simulink model "UAV_Hover_Sim_Soln"  (R2025a)
settings: Solver=VariableStepAuto  StartTime=0.0  StopTime=inf  RelTol=1e-3
undefined symbols (not defined in the file): quad_m, W
libraries: slpidlib x1, aerolibanimutils x1, uavutilslib x1, aerolibobsolete x1
settings Model: Creator=Aorus PC  LastModifiedBy=esmithzb
settings OptimizationCC: ReuseModelBlockBuffer=off
settings DebuggingCC: UnderspecifiedInitializationDetection=Classic  MergeDetectMultiDrivingBlocksExec=none
settings ModelReferenceCC: PropagateSignalLabelsOutOfModel=off
settings RTWCC: GPUComputeCapability=3.5

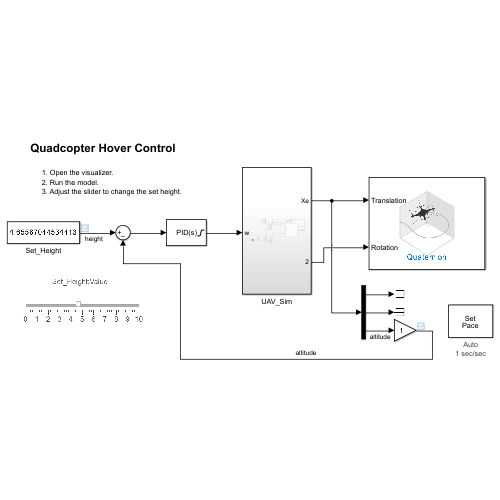
[thumbnail: Simulink's stored preview of the top-level diagram]
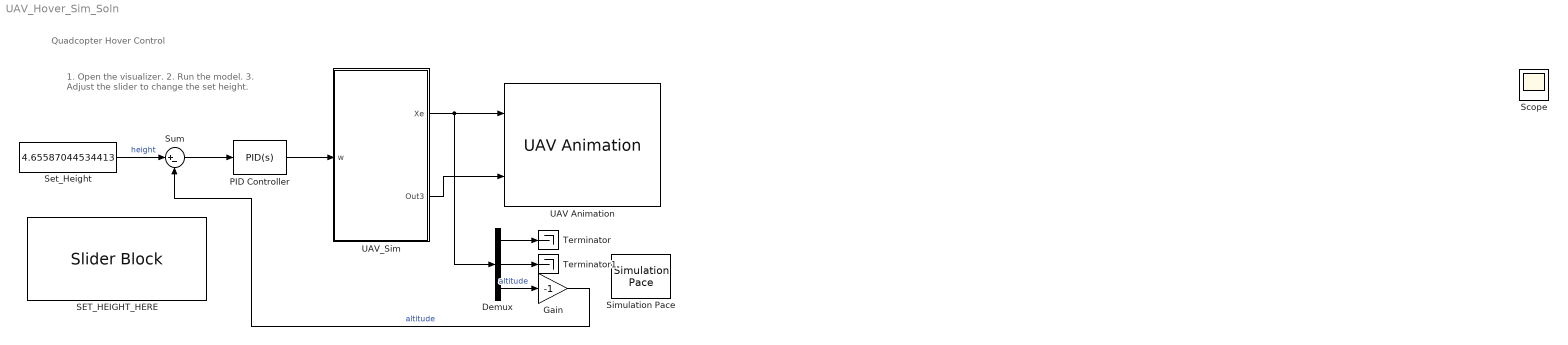
== system UAV_Hover_Sim_Soln ==
  note: 1. Open the visualizer.
      | 2. Run the model.
      | 3. Adjust the slider to change the set height.
  note: Quadcopter Hover Control
  Demux : Demux  Outputs=3
  Gain : Gain  Gain=-1
  PID Controller : slpidlib/PID Controller  Controller=PID  Form=Parallel  TimeDomain=Continuous-time  UseExternalTs=off  SampleTime=-1  IntegratorMethod=Forward Euler  FilterMethod=Forward Euler  ControllerParametersSource=internal  P=17.0862146274148  I=0.608175767121999  UseKiTs=off  D=103.307761768291  UseExternalDerivativeSource=off  N=1.18940326833611  UseFilter=on  TunerSelectOption=Transfer Function Based (PID Tuner App)  InitialConditionSource=internal  InitialConditionForIntegrator=4000  InitialConditionForFilter=0  DifferentiatorICPrevScaledInput=0  ExternalReset=none  TrackingMode=off  Kt=1  LimitOutput=on  SatLimitsSource=internal  UpperSaturationLimit=1e4  LowerSaturationLimit=0  LinearizeAsGain=on  AntiWindupMode=back-calculation  Kb=1  LimitIntegrator=on  UpperIntegratorSaturationLimit=1e4  LowerIntegratorSaturationLimit=0  POutMin=[]  POutMax=[]  IOutMin=[]  IOutMax=[]  DOutMin=[]  DOutMax=[]  NOutMin=[]  NOutMax=[]  SumOutMin=[]  SumOutMax=[]  SaturationOutMin=[]  SaturationOutMax=[]  PParamMin=[]  PParamMax=[]  IParamMin=[]  IParamMax=[]  DParamMin=[]  DParamMax=[]  NParamMin=[]  NParamMax=[]  KbParamMin=[]  KbParamMax=[]  KtParamMin=[]  KtParamMax=[]  KbOutMin=[]  KbOutMax=[]  KtOutMin=[]  KtOutMax=[]  IntegratorOutMin=[]  IntegratorOutMax=[]  FilterOutMin=[]  FilterOutMax=[]  SumI1OutMin=[]  SumI1OutMax=[]  SumI2OutMin=[]  SumI2OutMax=[]  SumI3OutMin=[]  SumI3OutMax=[]  SumI4OutMin=[]  SumI4OutMax=[]  SumDOutMin=[]  SumDOutMax=[]  DifferentiatorOutMin=[]  DifferentiatorOutMax=[]  FilterDiffOutCoefMin=[]  FilterDiffOutCoefMax=[]  ReciprocalOutMin=[]  ReciprocalOutMax=[]  SumDenOutMin=[]  SumDenOutMax=[]  SumNumOutMin=[]  SumNumOutMax=[]  DivideOutMin=[]  DivideOutMax=[]  UdiffTsProdOutMin=[]  UdiffTsProdOutMax=[]  NTsProdOutMin=[]  NTsProdOutMax=[]  UintegralTsProdOutMin=[]  UintegralTsProdOutMax=[]  UngainTsProdOutMin=[]  UngainTsProdOutMax=[]  ClampingZeroOutDataTypeStr=Inherit: Inherit via back propagation  ClampingZeroOutMin=[]  ClampingZeroOutMax=[]  FilterDenConstantOutDataTypeStr=Inherit: Inherit via back propagation  FilterDenConstantOutMin=[]  FilterDenConstantOutMax=[]  PCopyOutDataTypeStr=Inherit: Inherit via back propagation  PCopyOutMin=[]  PCopyOutMax=[]  NCopyOutDataTypeStr=Inherit: Inherit via back propagation  NCopyOutMin=[]  NCopyOutMax=[]  IntegratorContinuousStateAttributes=''  IntegratorStateMustResolveToSignalObject=off  IntegratorRTWStateStorageClass=Auto  FilterContinuousStateAttributes=''  FilterStateMustResolveToSignalObject=off  FilterRTWStateStorageClass=Auto  ParallelPVariant=InternalParameters  IdealPVariant=Disabled  IVariant=InternalParameters  DVariant=InternalParameters  IntegratorVariant=Continuous  SatVariant=Enabled  AWVariant=BackCalculation  PCopyVariant=Disabled  TRVariant=Disabled  FdbkBlocksVariant=Forward  IdealPFdbkVariant=Disabled  SatFdbkVariant=Disabled  DerivativeFilterVariant=ContFilter  NVariant=InternalParameters  NCopyVariant=Disabled  FilterICVariant=InternalICsFilter  IntegratorICVariant=InternalICs  ExternalResetVariant=Disabled  TRSumVariant=Passthrough  SumFdbkVariant=Disabled  SumVariant=Sum_PID  TsampFilterVariant=InternalTs  TsampNgainVariant=Passthrough  TsampIntegralVariant=Disabled_SignalSpec  ExternalSaturationOutDataTypeStr=Inherit: Same as second input  DerivativeSourceVariant=ErrorSignal  PreIntVariant=InternalPreInt
  SET_HEIGHT_HERE : SliderBlock  ScaleMax=10  TickInterval=1
  Set_Height : Constant  Value=4.65587044534413
  Simulation Pace : aerolibanimutils/Simulation Pace  SimulationPace=1  SleepMode=Auto  OutputPaceError=off  SampleTime=1/30
  Sum : Sum  Inputs=|+-
  Terminator : Terminator
  Terminator1 : Terminator
  UAV Animation : uavutilslib/UAV Animation  NumUAV=1  DynamicUAVConfig=off  UAVType=Multirotor  UAVSize=4  UAVColor=[1 0 0]  UAVTrajectoryAlpha=1  InertialZDirection=Down  RotationFormat=Quaternion  DrawMarkers=off  SampleTime=-1
  UAV_Sim : Subsystem
  Scope : Scope
      settings: TimeSpan=20  ActiveDisplayYMinimum=0  ActiveDisplayYMaximum=12  YLabel=Altitude (m)
  wires:
  UAV_Sim/1(Xe) -> Demux/1, UAV Animation/1
  UAV_Sim/2(Out3) -> UAV Animation/2
  Demux/1 -> Terminator/1
  Demux/2 -> Terminator1/1
  Gain/1 -> Sum/2  "altitude"
  Set_Height/1 -> Sum/1  "height"
  Demux/3 -> Gain/1  "altitude"
  PID Controller/1 -> UAV_Sim/1(w)
  Sum/1 -> PID Controller/1

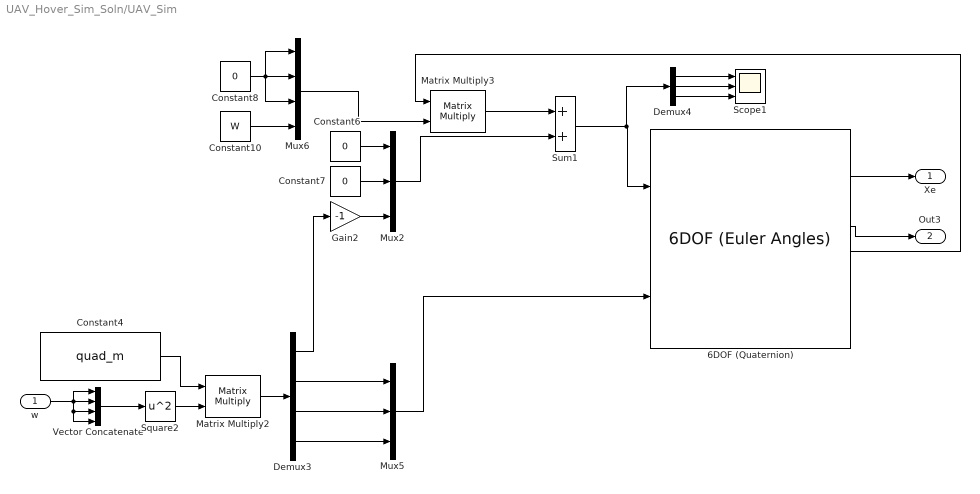
== system UAV_Hover_Sim_Soln/UAV_Sim ==
  w : Inport
  6DOF (Quaternion) : aerolibobsolete/6DOF (Euler Angles)  units=Metric (MKS)  mtype=Fixed  rep=Quaternion  xme_0=[0 0 0]  Vm_0=[0 0 0]  eul_0=[0 0 0]  pm_0=[0 0 0]  mass_0=1.0  mass_e=0.5  mass_f=2.0  inertia=eye(3)  inertia_e=eye(3)  inertia_f=2*eye(3)  k_quat=1.0  vre_flag=off  abi_flag=off  aMode=0  xme_statename=''  Vm_statename=''  eul_statename=''  quat_statename=''  pm_statename=''  mass_statename=''
  Constant10 : Constant  Value=W
  Constant4 : Constant  Value=quad_m
  Constant6 : Constant  Value=0
  Constant7 : Constant  Value=0
  Constant8 : Constant  Value=0
  Demux3 : Demux
  Demux4 : Demux  Outputs=3
  Gain2 : Gain  Gain=-1
  Matrix Multiply2 : Product  Multiplication=Matrix(*)
  Matrix Multiply3 : Product  Multiplication=Matrix(*)
  Mux2 : Mux  Inputs=3
  Mux5 : Mux  Inputs=3
  Mux6 : Mux
  Scope1 : Scope  NumInputPorts=3
      settings: ActiveDisplayYMinimum=-7E-15  ActiveDisplayYMaximum=8E-16  DataLoggingVariableName=ScopeData2
  Square2 : Math  Operator=square
  Sum1 : Sum
  Vector Concatenate : Concatenate  NumInputs=4
  Xe : Outport
  Out3 : Outport  Port=2
  wires:
  Mux2/1 -> Sum1/2
  Matrix Multiply3/1 -> Sum1/1
  Demux4/1 -> Scope1/1
  Mux6/1 -> Matrix Multiply3/2
  Constant10/1 -> Mux6/4
  Sum1/1 -> 6DOF (Quaternion)/1, Demux4/1
  Demux4/2 -> Scope1/2
  Constant4/1 -> Matrix Multiply2/1
  Demux3/1 -> Gain2/1
  Mux5/1 -> 6DOF (Quaternion)/2
  Square2/1 -> Matrix Multiply2/2
  Matrix Multiply2/1 -> Demux3/1
  Demux3/2 -> Mux5/1
  Demux3/3 -> Mux5/2
  Demux3/4 -> Mux5/3
  Constant8/1 -> Mux6/1, Mux6/3, Mux6/2
  Constant6/1 -> Mux2/1
  Constant7/1 -> Mux2/2
  Gain2/1 -> Mux2/3
  Demux4/3 -> Scope1/3
  w/1 -> Vector Concatenate/4, Vector Concatenate/3, Vector Concatenate/1, Vector Concatenate/2
  6DOF (Quaternion)/4 -> Out3/1
  6DOF (Quaternion)/5 -> Matrix Multiply3/1
  6DOF (Quaternion)/2 -> Xe/1
  Vector Concatenate/1 -> Square2/1
